simulink model "example_simulink_send_receive"  (R2019a)
settings: Solver=FixedStepAuto  StartTime=0.0  StopTime=inf  FixedStep=1/75  RelTol=1e-3  EnableMultiTasking=on
undefined symbols (not defined in the file or in its folder): CR, LF
libraries: instrumentlib x3, etargetslib x1, aerolibanimutils x1
settings Model: Creator=marcell  LastModifiedBy=marcellmocher
settings DataIOCC: LimitDataPoints=on  ReturnWorkspaceOutputs=off
settings OptimizationCC: LifeSpan=inf
settings DebuggingCC: AllowSymbolicDim=off  SFUnexpectedBacktrackingDiag=warning  SFNoUnconditionalDefaultTransitionDiag=warning  SFExecutionAtInitializationDiag=none  ArithmeticOperatorsInVariantConditions=warning
settings ModelReferenceCC: PropagateSignalLabelsOutOfModel=off
settings SFSimCC: SimUseLocalCustomCode=off
settings RTWCC: RTWUseLocalCustomCode=off
settings CodeAppCC: StateflowObjectComments=on
settings GRTTargetCC: TargetLangStandard=C89/C90 (ANSI)
settings ConfigComp: CovMetricSettings=dw  CovHtmlReporting=on  CovSaveCumulativeToWorkspaceVar=on  CovSaveSingleToWorkspaceVar=on  CovExternalEMLEnable=off

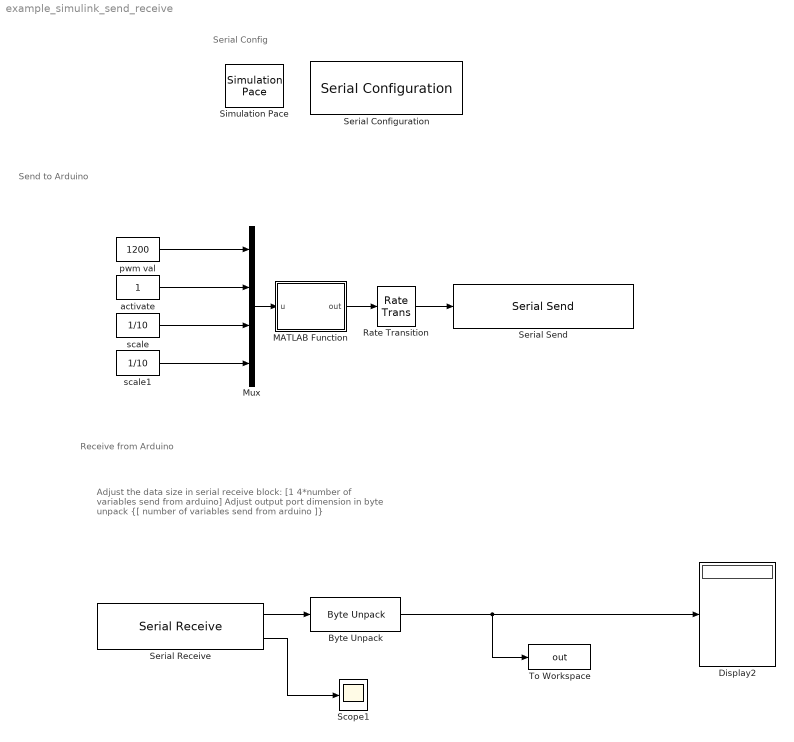
== system example_simulink_send_receive ==
  note: Adjust the data size in serial receive block: [1 4*number of variables send from arduino]
      | Adjust output port dimension in byte unpack {[ number of variables send from arduino ]}
  note: Send to Arduino
  note: Serial Config
  note: Receive from Arduino
  Byte Unpack : etargetslib/Byte Unpack  dimensions={[4]}  datatypes={'single'}  byteAlign=1
      settings: SourceProductName=MATLAB Coder
  Display2 : Display
  MATLAB Function : MATLAB Function  TreatAsAtomicUnit=on
  Mux : Mux  Inputs=[1 1 1 1]
  Rate Transition : RateTransition  OutPortSampleTime=1/75
  Scope1 : Scope
  Serial Configuration : instrumentlib/Serial Configuration  Priority=-200000  ComPortMenu=<Please select a port...>  ComPort=<Please select a port...>  BaudRate=115200  DataBits=8  Parity=none  StopBits=1  FlowControl=none  Timeout=10  ByteOrder=LittleEndian
  "Serial Receive " : instrumentlib/Serial Receive  ComPortMenu=<Please select a port...>  ComPort=<Please select a port...>  Header=aaaaaaaa  Terminator=CR/LF ('\r\n')  DataSize="[1  16]"  DataType=uint8  EnableBlockingMode=off  ActionDataUnavailable=Output last received value  CustomValue=0  SampleTime=1/75  mask(Serial Receive){}
  Serial Send : instrumentlib/Serial Send  ComPortMenu=<Please select a port...>  ComPort=<Please select a port...>  Header=bbbb  Terminator=CR/LF ('\r\n')  EnableBlockingMode=on
  Simulation Pace : aerolibanimutils/Simulation Pace  SimulationPace=1  SleepMode=MATLAB Thread  OutputPaceError=off  SampleTime=1/75
  To Workspace : ToWorkspace  VariableName=out  SaveFormat=Structure With Time  SampleTime=-1
  activate : Constant  OutDataTypeStr=single
  "pwm val " : Constant  Value=1200  OutDataTypeStr=single
  scale : Constant  Value=1/10  OutDataTypeStr=single
  scale1 : Constant  Value=1/10  OutDataTypeStr=single
  wires:
  Rate Transition/1 -> Serial Send/1
  MATLAB Function/1(out) -> Rate Transition/1
  Mux/1 -> MATLAB Function/1(u)
  activate/1 -> Mux/2
  scale/1 -> Mux/3
  scale1/1 -> Mux/4
  "pwm val "/1 -> Mux/1
  "Serial Receive "/1 -> Byte Unpack/1
  Byte Unpack/1 -> To Workspace/1, Display2/1
  "Serial Receive "/2 -> Scope1/1

== matlab function example_simulink_send_receive/MATLAB Function ==
  data: u input; out output
% /%%
%%%%%%%%%%%%%%%%%%%%%%%%%%%%%%%%%%%%%%%%%%%%%%%%%%%%%%%%%%%%%%%%%%%%%%%%%%%%%%
% @file     
% @author   Marcell Mocher
% @version  V0.0.1
% @date     16.6.2016
% @brief    converts single input to byte array
%
%
%%%%%%%%%%%%%%%%%%%%%%%%%%%%%%%%%%%%%%%%%%%%%%%%%%%%%%%%%%%%%%%%%%%%%%%%%%%%%%
% @attention
%
%
%
%
%%%%%%%%%%%%%%%%%%%%%%%%%%%%%%%%%%%%%%%%%%%%%%%%%%%%%%%%%%%%%%%%%%%%%%%%%%%%%%
%/
function out = fcn(u)
u_single = single(u);
u_byte = typecast(u_single,'uint8');
len_single = uint8(numel(u_single));
len_byte = uint8(numel(u_byte));
y = uint8(zeros((len_single*4)+1,1));
y(1) = len_byte;
for i = 1:len_byte
   y(i+1) = u_byte(i) ;
end
out = y;
